simulink model "ponto3"  (R2016b)
settings: Solver=VariableStepAuto  StartTime=0.0  StopTime=100  RelTol=1e-3
values from neighbouring files (symbols this model uses):
  ah = [xu xw -aa0*u0 -g*cos(tt0) 0 ... (first row only)    [tb30.m]
  bh = [xde xdt; zde 0; mde+mwp*zde mdt; 0 0; 0 0]    [tb30.m]
  f = ([1 0 0 0 0;0 0 0 0 1]*g)^-1    [tb30.m]
  k2 = lqr(ah,bh,q,r)    [tb30.m]
settings Model: Creator=inespassinhas  LastModifiedBy=inespassinhas

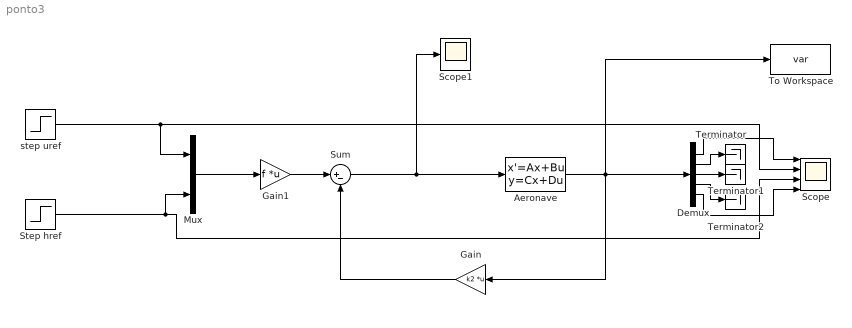
== system ponto3 ==
  Aeronave : StateSpace  A=ah  B=bh  C=eye(5)  D=zeros(5,2)  X0=[0 0 0 0 200]
  Demux : Demux  Outputs=5
  Gain : Gain  Gain=k2  Multiplication=Matrix(K*u)
  Gain1 : Gain  Gain=f  Multiplication=Matrix(K*u)
  Mux : Mux  Inputs=2
  Scope : Scope  NumInputPorts=4
  Scope1 : Scope
  Step href : Step  Time=50  Before=200  After=210  SampleTime=0
  Sum : Sum  Inputs=|+-
  Terminator : Terminator
  Terminator1 : Terminator
  Terminator2 : Terminator
  To Workspace : ToWorkspace  VariableName=var  SaveFormat=Structure With Time  SampleTime=-1
  step uref : Step  Time=5  After=4  SampleTime=0
  wires:
  Gain/1 -> Sum/2
  Aeronave/1 -> Gain/1, Demux/1, To Workspace/1
  Sum/1 -> Scope1/1, Aeronave/1
  step uref/1 -> Mux/1, Scope/2
  Step href/1 -> Scope/3, Mux/2
  Mux/1 -> Gain1/1
  Gain1/1 -> Sum/1
  Demux/1 -> Scope/1
  Demux/5 -> Scope/4
  Demux/2 -> Terminator/1
  Demux/4 -> Terminator2/1
  Demux/3 -> Terminator1/1
